simulink model "task8_v23"  (R2023b)
settings: Solver=VariableStepAuto  StartTime=0.0  StopTime=10.0  RelTol=1e-3
model workspace (MAT data in the model file):
  SampleTime = 1
libraries: robotcorelib x2, robotmaniplib x1
settings Model: Creator=Nico  LastModifiedBy=Nico
settings RTWCC: GPUComputeCapability=5.0

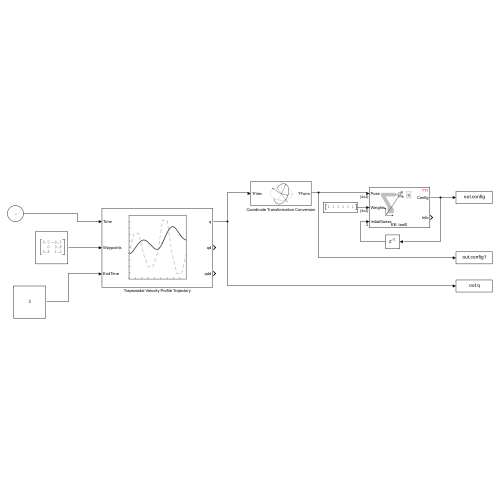
[thumbnail: Simulink's stored preview of the top-level diagram]
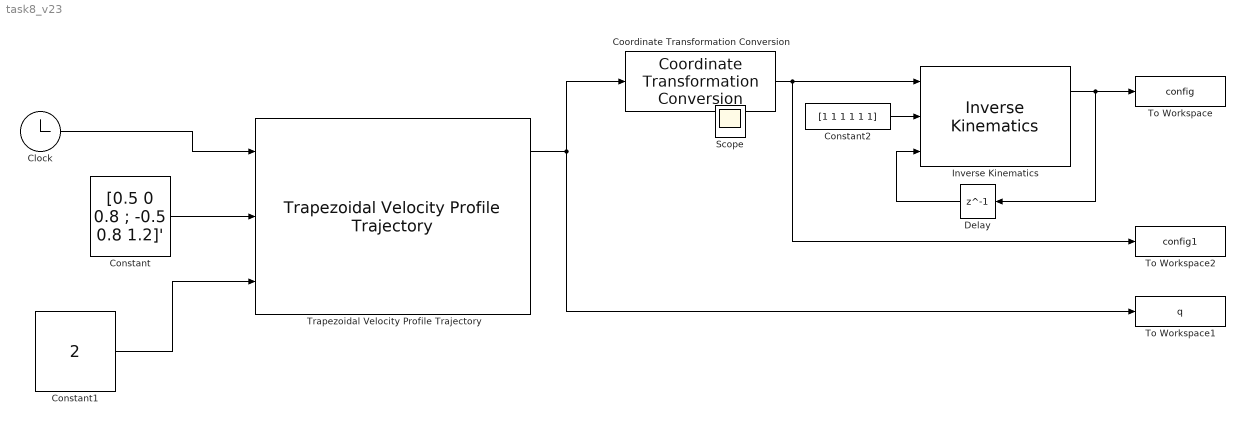
== system task8_v23 ==
  Clock : Clock
  Constant : Constant  Value=[0.5 0 0.8 ; -0.5 0.8 1.2]'
  Constant1 : Constant  Value=2
  Constant2 : Constant  Value=[1 1 1 1 1 1]
  Coordinate Transformation Conversion : robotcorelib/Coordinate Transformation Conversion  InputRepresentation=Translation Vector  InputEulerSequence=ZYX  ShowTrVecInputPort=on  OutputRepresentation=Homogeneous Transformation  OutputEulerSequence=ZYX  ShowTrVecOutputPort=on  SimulateUsing=Interpreted execution
  Delay : Delay  DelayLength=1  InitialCondition=0
  Inverse Kinematics : robotmaniplib/Inverse Kinematics  RigidBodyTree=robotRBT  EndEffector=tool0  ShowInfo=on  SolverName=BFGS Gradient Projection  EnforceJointLimits=on  MaxIterations=1500  MaxTime=10  GradientTolerance=1e-7  SolutionTolerance=1e-6  StepTolerance=1e-14  ErrorChangeTolerance=1e-12  UseErrorDamping=on  DampingBias=0.0025  SimulateUsing=Interpreted execution
  To Workspace : ToWorkspace  VariableName=config  SampleTime=-1
  To Workspace1 : ToWorkspace  VariableName=q  SampleTime=-1
  To Workspace2 : ToWorkspace  VariableName=config1  SampleTime=-1
  Trapezoidal Velocity Profile Trajectory : robotcorelib/Trapezoidal Velocity Profile Trajectory  WaypointSource=External  Waypoints=[ 0, -0.5, -1; 0, 0.5, 1 ]  NumParams=1  Parameter1=End Time  Parameter2=End Time  ParameterSource=External  PeakVelocity=[ 2; 2 ]  Acceleration=[ 1; 2 ]  EndTime=[ 1; 1 ]  AccelTime=[ 1; 2 ]  SimulateUsing=Interpreted execution
  Scope : Scope
  wires:
  Clock/1 -> Trapezoidal Velocity Profile Trajectory/1
  Constant/1 -> Trapezoidal Velocity Profile Trajectory/2
  Trapezoidal Velocity Profile Trajectory/1 -> Coordinate Transformation Conversion/1, To Workspace1/1
  Coordinate Transformation Conversion/1 -> Inverse Kinematics/1, To Workspace2/1
  Inverse Kinematics/1 -> Delay/1, To Workspace/1
  Constant1/1 -> Trapezoidal Velocity Profile Trajectory/3
  Constant2/1 -> Inverse Kinematics/2
  Delay/1 -> Inverse Kinematics/3
